simulink model "FuelCell2"  (R2016b)
settings: Solver=ode45  StartTime=0.0  StopTime=10.0  RelTol=1e-3
undefined symbols (not defined in the file): A, B, C, J, Jmax, lam, n, Rc, Tr
libraries: simulink x1
settings Model: Creator=Kelly  LastModifiedBy=Kelly

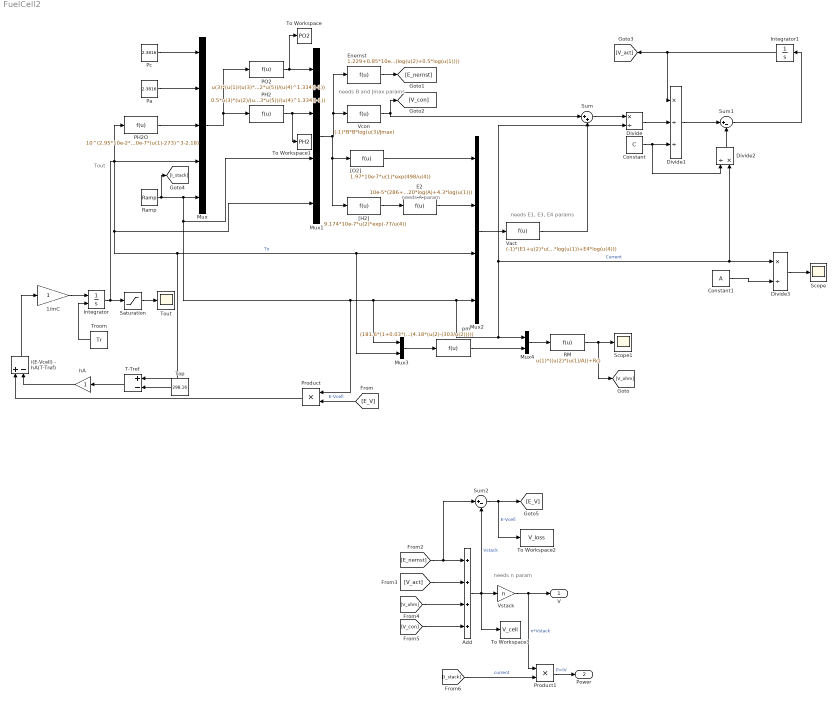
== system FuelCell2 ==
  note: Tout
  note: needs E1, E3, E4 params
  note: needs B and Jmax params
  note: needs A param
  note: needs n param
  1/mC : Gain
  Add : Sum  Inputs=4
  Constant : Constant  Value=C
  Constant1 : Constant  Value=A
  Divide : Product  Inputs=*/
  Divide1 : Product  Inputs=*//
  Divide2 : Product  Inputs=/*
  Divide3 : Product  Inputs=*/
  E2 : Fcn  Expr=10e-5*(286+20*log(A)+4.3*log(u(1)))
  Enernst : Fcn  Expr=1.229+0.85*10e-3*(u(4)-298.15)+4.3085*10e-5*(log(u(2)+0.5*log(u(1))))
  Integrator : Integrator  InitialConditionSource=external
  Integrator1 : Integrator
  Mux : Mux  Inputs=5
  Mux1 : Mux
  Mux2 : Mux
  Mux3 : Mux  Inputs=2
  Mux4 : Mux  Inputs=2
  PH2 : Fcn  Expr=0.5*u(3)*(u(2)/(u(3)*exp((1.653*u(5))/(u(4)^1.334))-1))
  PH2O : Fcn  Expr=10^(2.95*10e-2*(u(1)-273)-9.18*10e-5*(u(1)-273)^2+1.44*10e-7*(u(1)-273)^3-2.18)
  PO2 : Fcn  Expr=u(3)*(u(1)/(u(3)*exp((4.192*u(5))/(u(4)^1.334))-1))
  Pa : Constant  Value=2.3816
  Pc : Constant  Value=2.3816
  Product : Product
  Product1 : Product
  RM : Fcn  Expr=u(1)*((u(2)*(u(1)/A))+Rc)
  Ramp : simulink/Sources/Ramp  slope=Jmax*A/100  start=0  X0=J*A/100
  Saturation : Saturate
  Scope : Scope
  Scope1 : Scope
  Sum : Sum  Inputs=|++
  Sum1 : Sum  Inputs=|+-
  Sum2 : Sum  Inputs=|+-
  T-Tref : Sum  Inputs=+-
  To Workspace : ToWorkspace  VariableName=PO2  SaveFormat=Timeseries  SampleTime=-1
  To Workspace1 : ToWorkspace  VariableName=PH2  SaveFormat=Timeseries  SampleTime=-1
  To Workspace2 : ToWorkspace  VariableName=V_loss  SaveFormat=Timeseries  SampleTime=-1
  To Workspace3 : ToWorkspace  VariableName=V_cell  SaveFormat=Timeseries  SampleTime=-1
  Top : Constant  Value=298.16
  Tout : Scope
  Troom : Constant  Value=Tr
  Vact : Fcn  Expr=(-1)*(E1+u(2)*u(3)+E3*u(3)*log(u(1))+E4*log(u(4)))
  Vcon : Fcn  Expr=(-1)*B*B*log(u(3)/Jmax)
  Vstack : Gain  Gain=n
  "[H2]" : Fcn  Expr=9.174*10e-7*u(2)*exp(-77/u(4))
  "[O2]" : Fcn  Expr=1.97*10e-7*u(1)*exp(498/u(4))
  hA : Gain
  i(E-Vcell) - hA(T-Tref) : Sum  Inputs=+-
  pm : Fcn  Expr=(181.6*(1+0.03*(u(1)/A)+0.062*(u(2)/303)*(u(1)/A)^2.5))/((lam-0.634-3*(u(1)/A))*exp(4.18*(u(2)-(303/u(2)))))
  V : Outport
  Power : Outport  Port=2
  wires:
  Pc/1 -> Mux/1
  Pa/1 -> Mux/2
  PH2O/1 -> Mux/3
  Integrator/1 -> T-Tref/1, Mux3/2, Mux2/3, Mux1/4, PH2O/1, Mux/4, Saturation/1  "To"
  Ramp/1 -> [I_stack], Product/1, Mux3/1, Divide2/2, Divide3/1, Divide/2, Mux4/1, Mux2/4, Mux1/3, Mux/5  "Current"
  Mux/1 -> PH2/1, PO2/1
  PO2/1 -> To Workspace/1, Mux1/1
  PH2/1 -> To Workspace1/1, Mux1/2
  Mux1/1 -> "[H2]"/1, "[O2]"/1, Vcon/1, Enernst/1
  "[H2]"/1 -> E2/1
  "[O2]"/1 -> Mux2/1
  E2/1 -> Mux2/2
  Mux2/1 -> Vact/1
  Vcon/1 -> [V_con], Sum/1
  [V_con] -> Add/4
  [V_ohm] -> Add/3
  [V_act] -> Add/2
  [E_nernst] -> Sum2/1, Add/1
  Add/1 -> To Workspace3/1, Sum2/2, Vstack/1  "Vstack"
  Vstack/1 -> Product1/1, V/1  "n*Vstack"
  Product1/1 -> Power/1  "P=IV"
  [I_stack] -> Product1/2  "current"
  Sum2/1 -> To Workspace2/1, [E_V]  "E-Vcell"
  [E_V] -> Product/2  "E-Vcell"
  Top/1 -> T-Tref/2
  T-Tref/1 -> hA/1
  hA/1 -> i(E-Vcell) - hA(T-Tref)/2
  Product/1 -> i(E-Vcell) - hA(T-Tref)/1
  i(E-Vcell) - hA(T-Tref)/1 -> 1/mC/1
  1/mC/1 -> Integrator/1
  Troom/1 -> Integrator/2
  Saturation/1 -> Tout/1
  Mux3/1 -> pm/1
  pm/1 -> Mux4/2
  Mux4/1 -> RM/1
  RM/1 -> [V_ohm], Scope1/1
  Enernst/1 -> [E_nernst]
  Vact/1 -> Sum/2
  Sum/1 -> Divide/1
  Divide/1 -> Divide1/2
  Constant/1 -> Divide2/1, Divide1/3
  Divide1/1 -> Sum1/1
  Divide2/1 -> Sum1/2
  Constant1/1 -> Divide3/2
  Divide3/1 -> Scope/1
  Sum1/1 -> Integrator1/1
  Integrator1/1 -> Divide1/1, [V_act]
